simulink model "hpt_frt_full"  (R2025a)
settings: Solver=ode23tb  StartTime=0.0  StopTime=0.6  RelTol=1e-3
undefined symbols (not defined in the file or in its folder): D11, Delta
libraries: spsThreePhaseVIMeasurementLib x3, spsLinearTransformerLib x3, spsSeriesRLCBranchLib x2, spsThreePhaseSeriesRLCBranchLib x2, spsThreePhaseTransformerTwoWindingsLib x2, spsUniversalBridgeLib x2, spsIGBTLib x1, spsThreePhaseProgrammableVoltageSourceLib x1, spsThreePhaseFaultLib x1, spsThreePhaseSeriesRLCLoadLib x1, spsVoltageMeasurementLib x1, spspowerguiLib x1
settings Model: Creator=m1391  LastModifiedBy=m1391

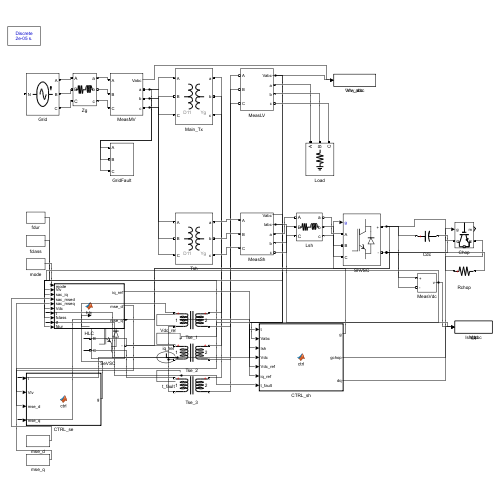
[thumbnail: Simulink's stored preview of the top-level diagram]
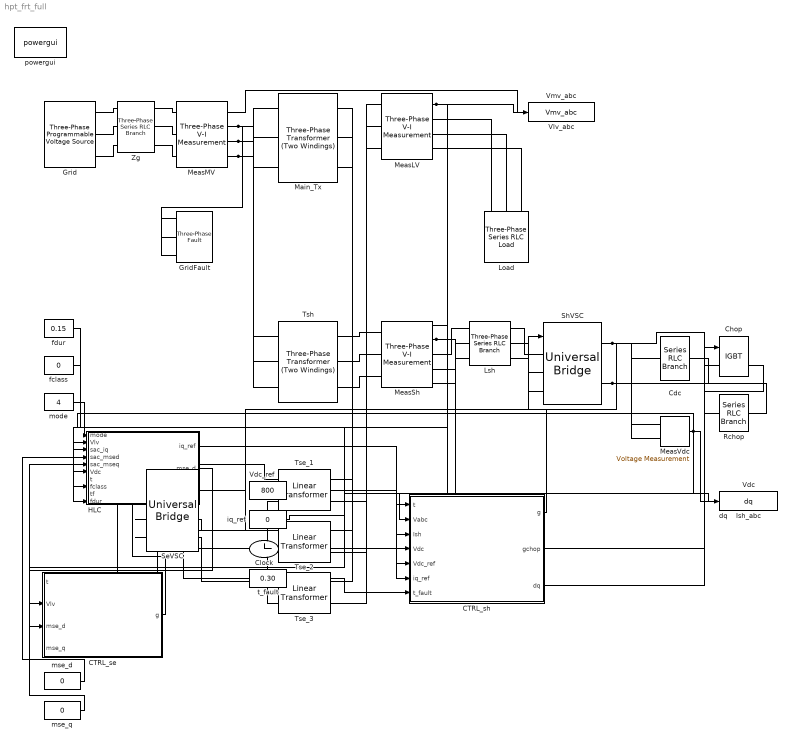
== system hpt_frt_full ==
  CTRL_se : MATLAB Function  TreatAsAtomicUnit=on
  CTRL_sh : MATLAB Function  TreatAsAtomicUnit=on
  Cdc : spsSeriesRLCBranchLib/Series RLC Branch  LConnTagsString=__new0  RConnTagsString=__new0  BranchType=C  Resistance=1  Inductance=1e-3  SetiL0=off  InitialCurrent=0  Capacitance=0.0022  Setx0=on  InitialVoltage=800  Measurements=None
  Chop : spsIGBTLib/IGBT  Ron=0.001  Lon=0  Vf=1  Tf=1e-6  Tt=2e-6  IC=0  Rs=1e5  Cs=inf  Measurements=on
  Clock : Clock
  Grid : spsThreePhaseProgrammableVoltageSourceLib/Three-Phase Programmable Voltage Source  PositiveSequence=[11250 0 50]  VariationEntity=None  VariationType=Table of time-amplitude pairs  VariationTypeAlt=Step  VariationStep=0.5  VariationRate=10  VariationMagnitude=0.3  VariationFrequency=2  VariationTiming=[1 2]  VariationPhaseA=off  Amplitudes=[1 0.8 1.2 1.0]  TimeValues=[0 0.1 0.15 0.2]  HarmonicGeneration=off  HarmonicA=[3 0.2 -25 0]  HarmonicB=[2 0.15 35 2]  Timing="[0.05  3]"  BusType=swing  Pref=0  Qref=0  Qmin=-inf  Qmax=inf
  GridFault : spsThreePhaseFaultLib/Three-Phase Fault  InitialStates=0  FaultA=off  FaultB=off  FaultC=off  GroundFault=off  SwitchTimes=[99 100]  External=off  SwitchStatus=NaN  FaultResistance=1  GroundResistance=0.01  SnubberResistance=1e6  SnubberCapacitance=inf  Measurements=None
  HLC : MATLAB Function  TreatAsAtomicUnit=on
  Ish_abc : ToWorkspace  VariableName=Ish_abc  SampleTime=2e-05
  Load : spsThreePhaseSeriesRLCLoadLib/Three-Phase Series RLC Load  LConnTagsString=A|B|C  Configuration=Y (grounded)  NominalVoltage=400  Vabc=[1e3 1e3 1e3]  Vabcp=[1e3 1e3 1e3]  NominalFrequency=50  UnbalancedPower=off  ActivePower=400000  InductivePower=0  CapacitivePower=0  Pabc=[10e3 9e3 11e3]  QLabc=[100 90 110]  QCabc=[100 90 110]  Pabcp=[10e3 9e3 11e3]  QLabcp=[100 90 110]  QCabcp=[100 90 110]  Measurements=None  LoadType=constant Z
  Lsh : spsThreePhaseSeriesRLCBranchLib/Three-Phase Series RLC Branch  LConnTagsString=A|B|C  RConnTagsString=A|B|C  BranchType=RL  Resistance=0.05  Inductance=0.003  Capacitance=1e-6  Measurements=None
  Main_Tx : spsThreePhaseTransformerTwoWindingsLib/Three-Phase Transformer (Two Windings)  Winding1Connection=Delta (D11)  Winding2Connection=Yg  CoreType=Three single-phase transformers  SetSaturation=off  Hysteresis=off  DataFile='hysteresis'  SetInitialFlux=off  Measurements=None  UNITS=pu  NominalPower=[400000,50]  Winding1=[10000,0.005,0.025]  Winding2=[400,0.005,0.025]  Rm=500  Lm=500  L0=0.5  Saturation=[ 0,0 ; 0.0024,1.2 ; 1.0,1.52 ]  InitialFluxes=[ 0.8 , -0.8 , 0.7 ]  BreakLoop=off  DiscreteSolver=Trapezoidal iterative  DataType=off  TransfoNumber=1
  MeasLV : spsThreePhaseVIMeasurementLib/Three-Phase V-I Measurement  VoltageMeasurement=phase-to-ground  SetLabelV=off  LabelV=Vabc  Vpu=off  VpuLL=off  CurrentMeasurement=no  SetLabelI=off  LabelI=Iabc  Ipu=off  Pbase=100e6  Vbase=500e3  OutputType=Complex  PhasorSimulation=off  PSBequivalent=0
  MeasMV : spsThreePhaseVIMeasurementLib/Three-Phase V-I Measurement  VoltageMeasurement=phase-to-ground  SetLabelV=off  LabelV=Vabc  Vpu=off  VpuLL=off  CurrentMeasurement=no  SetLabelI=off  LabelI=Iabc  Ipu=off  Pbase=100e6  Vbase=500e3  OutputType=Complex  PhasorSimulation=off  PSBequivalent=0
  MeasSh : spsThreePhaseVIMeasurementLib/Three-Phase V-I Measurement  VoltageMeasurement=phase-to-ground  SetLabelV=off  LabelV=Vabc  Vpu=off  VpuLL=off  CurrentMeasurement=yes  SetLabelI=off  LabelI=Iabc  Ipu=off  Pbase=100e6  Vbase=500e3  OutputType=Complex  PhasorSimulation=off  PSBequivalent=0
  MeasVdc : spsVoltageMeasurementLib/Voltage Measurement  PhasorSimulation=off  OutputType=Complex  PSBequivalent=0
  Rchop : spsSeriesRLCBranchLib/Series RLC Branch  LConnTagsString=__new0  RConnTagsString=__new0  BranchType=R  Resistance=5.3333  Inductance=1e-3  SetiL0=off  InitialCurrent=0  Capacitance=1e-6  Setx0=off  InitialVoltage=0  Measurements=None
  SeVSC : spsUniversalBridgeLib/Universal Bridge  Arms=3  SnubberResistance=1e5  SnubberCapacitance=inf  Device=IGBT / Diodes  Ron=1e-3  Lon=0  ForwardVoltages="[  0  0  ]"  ForwardVoltage=0  GTOparameters=[ 10e-6 , 20e-6 ]  IGBTparameters=[ 1e-6 , 2e-6 ]  Measurements=None  Measurements_2=None  converterType=Rectifier
  ShVSC : spsUniversalBridgeLib/Universal Bridge  Arms=3  SnubberResistance=1e5  SnubberCapacitance=inf  Device=IGBT / Diodes  Ron=1e-3  Lon=0  ForwardVoltages="[  0  0  ]"  ForwardVoltage=0  GTOparameters=[ 10e-6 , 20e-6 ]  IGBTparameters=[ 1e-6 , 2e-6 ]  Measurements=None  Measurements_2=None  converterType=Rectifier
  Tse_1 : spsLinearTransformerLib/Linear Transformer  UNITS=pu  NominalPower=[30000,50]  winding1=[400,0.002,0.03]  winding2=[46.2,0.002,0.03]  ThreeWindings=off  winding3=[ 315e3 0.002 0.08 ]  RmLm=[ 500 500 ]  Measurements=None  DataType=off
  Tse_2 : spsLinearTransformerLib/Linear Transformer  UNITS=pu  NominalPower=[30000,50]  winding1=[400,0.002,0.03]  winding2=[46.2,0.002,0.03]  ThreeWindings=off  winding3=[ 315e3 0.002 0.08 ]  RmLm=[ 500 500 ]  Measurements=None  DataType=off
  Tse_3 : spsLinearTransformerLib/Linear Transformer  UNITS=pu  NominalPower=[30000,50]  winding1=[400,0.002,0.03]  winding2=[46.2,0.002,0.03]  ThreeWindings=off  winding3=[ 315e3 0.002 0.08 ]  RmLm=[ 500 500 ]  Measurements=None  DataType=off
  Tsh : spsThreePhaseTransformerTwoWindingsLib/Three-Phase Transformer (Two Windings)  Winding1Connection=Delta (D11)  Winding2Connection=Yg  CoreType=Three single-phase transformers  SetSaturation=off  Hysteresis=off  DataFile='hysteresis'  SetInitialFlux=off  Measurements=None  UNITS=pu  NominalPower=[120000,50]  Winding1=[10000,0.005,0.02]  Winding2=[400,0.005,0.02]  Rm=500  Lm=500  L0=0.5  Saturation=[ 0,0 ; 0.0024,1.2 ; 1.0,1.52 ]  InitialFluxes=[ 0.8 , -0.8 , 0.7 ]  BreakLoop=off  DiscreteSolver=Trapezoidal iterative  DataType=off  TransfoNumber=1
  Vdc : ToWorkspace  VariableName=Vdc  SampleTime=2e-05
  Vdc_ref : Constant  Value=800
  Vlv_abc : ToWorkspace  VariableName=Vlv_abc  SampleTime=2e-05
  Vmv_abc : ToWorkspace  VariableName=Vmv_abc  SampleTime=2e-05
  Zg : spsThreePhaseSeriesRLCBranchLib/Three-Phase Series RLC Branch  LConnTagsString=A|B|C  RConnTagsString=A|B|C  BranchType=RL  Resistance=11.7851  Inductance=0.26259  Capacitance=1e-6  Measurements=None
  dq : ToWorkspace  VariableName=dq  SampleTime=2e-05
  fclass : Constant  Value=0
  fdur : Constant  Value=0.15
  iq_ref : Constant  Value=0
  mode : Constant  Value=4
  mse_d : Constant  Value=0
  mse_q : Constant  Value=0
  powergui : spspowerguiLib/powergui  Priority=1  SimulationMode=Discrete  SampleTime=2e-05  frequency=60  Iterations=50  frequencyindice=60  Pbase=100e6  ErrMax=1e-4  UnitsV=kV  UnitsW=MW  buscounter=0  FunctionMessages=off  echomessages=off  EnableUseOfTLC=off  CurrentSourceSwitches=off  DisableSnubberDevices=off  DisableRonSwitches=off  DisableVfSwitches=off  DisplayEquations=off  AutomaticDiscreteSolvers=off  SolverType=Tustin/Backward Euler (TBE)  Interpol=off  ExternalGateDelay=off  methode=off  Ts=100  x0status=blocks  SPID=on  SwTol=0  HookPort=off  NonlinearTolerance=1e-4  nMaxIteration=100  ContinueOnMaxIteration=off  RestoreLinks=warning  ResistiveCurrentMeasurement=off  Frange=[0:2:500]  Ylog=off  Xlog=on  ShowGrid=off  save=off  variable=ZData  structure=0  ZoomFFT=off  StartTime=0.0  cycles=1  DisplayStyle=1  fundamental=60  FreqAxis=off  MaxFrequency=1000  frequencyindicesteady=1  RmsSteady=1  display=off
  t_fault : Constant  Value=0.30
  wires:
  MeasMV/1 -> Vmv_abc/1
  MeasLV/1 -> Vlv_abc/1, CTRL_se/2(Vlv), HLC/2(Vlv)
  MeasSh/1 -> CTRL_sh/2(Vabc)
  MeasSh/2 -> CTRL_sh/3(Ish), Ish_abc/1
  MeasVdc/1 -> CTRL_sh/4(Vdc), Vdc/1, HLC/6(Vdc)
  Clock/1 -> CTRL_sh/1(t), CTRL_se/1(t), HLC/7(t)
  Vdc_ref/1 -> CTRL_sh/5(Vdc_ref)
  t_fault/1 -> CTRL_sh/7(t_fault), HLC/9(tf)
  CTRL_sh/1(g) -> ShVSC/1
  CTRL_sh/2(gchop) -> Chop/1
  CTRL_sh/3(dq) -> dq/1
  CTRL_se/1(g) -> SeVSC/1
  mode/1 -> HLC/1(mode)
  iq_ref/1 -> HLC/3(sac_iq)
  mse_d/1 -> HLC/4(sac_msed)
  mse_q/1 -> HLC/5(sac_mseq)
  fclass/1 -> HLC/8(fclass)
  fdur/1 -> HLC/10(fdur)
  HLC/1(iq_ref) -> CTRL_sh/6(iq_ref)
  HLC/2(mse_d) -> CTRL_se/3(mse_d)
  HLC/3(mse_q) -> CTRL_se/4(mse_q)
  connections:
  Grid/RConn1 -- Zg/LConn1
  Zg/RConn1 -- MeasMV/LConn1
  GridFault/LConn1 -- MeasMV/RConn1 -- Main_Tx/LConn1 -- Tsh/LConn1
  MeasLV/RConn1 -- Load/LConn1
  Grid/RConn2 -- Zg/LConn2
  Zg/RConn2 -- MeasMV/LConn2
  GridFault/LConn2 -- MeasMV/RConn2 -- Main_Tx/LConn2 -- Tsh/LConn2
  MeasLV/RConn2 -- Load/LConn2
  Grid/RConn3 -- Zg/LConn3
  Zg/RConn3 -- MeasMV/LConn3
  GridFault/LConn3 -- MeasMV/RConn3 -- Main_Tx/LConn3 -- Tsh/LConn3
  MeasLV/RConn3 -- Load/LConn3
  Tsh/RConn1 -- MeasSh/LConn1
  MeasSh/RConn1 -- Lsh/LConn1
  Lsh/RConn1 -- ShVSC/LConn1
  Tsh/RConn2 -- MeasSh/LConn2
  MeasSh/RConn2 -- Lsh/LConn2
  Lsh/RConn2 -- ShVSC/LConn2
  Tsh/RConn3 -- MeasSh/LConn3
  MeasSh/RConn3 -- Lsh/LConn3
  Lsh/RConn3 -- ShVSC/LConn3
  Cdc/LConn1 -- ShVSC/RConn1 -- MeasVdc/LConn1 -- Chop/LConn1 -- SeVSC/RConn1
  Cdc/RConn1 -- MeasVdc/LConn2 -- Rchop/RConn1 -- ShVSC/RConn2 -- SeVSC/RConn2
  Chop/RConn1 -- Rchop/LConn1
  Main_Tx/RConn1 -- Tse_1/RConn1
  Tse_1/RConn2 -- MeasLV/LConn1
  Main_Tx/RConn2 -- Tse_2/RConn1
  Tse_2/RConn2 -- MeasLV/LConn2
  Main_Tx/RConn3 -- Tse_3/RConn1
  Tse_3/RConn2 -- MeasLV/LConn3
  SeVSC/LConn1 -- Tse_1/LConn1
  SeVSC/LConn2 -- Tse_2/LConn1
  SeVSC/LConn3 -- Tse_3/LConn1
  Tse_2/LConn2 -- Tse_1/LConn2 -- Tse_3/LConn2

== matlab function hpt_frt_full/CTRL_se ==
  data: t input; g output; Vlv input; mse_d input; mse_q input
function g = ctrl(t, Vlv, mse_d, mse_q)
%#codegen
persistent th wint tprev
if isempty(th) || t<1e-9; th=0; wint=0; tprev=0; end
dt=t-tprev; if dt<0;dt=0;end; if dt>1e-3;dt=1e-3;end; tprev=t;
w0=2*pi*50;
Va=Vlv(1); Vb=Vlv(2); Vc=Vlv(3);
Valpha=(2/3)*(Va-0.5*Vb-0.5*Vc); Vbeta=(2/3)*(sqrt(3)/2)*(Vb-Vc);
Vd= cos(th)*Valpha+sin(th)*Vbeta; Vq=-sin(th)*Valpha+cos(th)*Vbeta;
Vm=sqrt(Vd*Vd+Vq*Vq); if Vm<50;Vm=50;end
wint=wint+1500*(Vq/Vm)*dt; if wint>150;wint=150;elseif wint<-150;wint=-150;end
w=w0+90*(Vq/Vm)+wint; th=th+w*dt; th=mod(th,2*pi);
% map SAC m_se (pu of LV phase, +/-0.2) -> VSC modulation index (+/-1): K=5
md=5*mse_d; mq=5*mse_q;
ma=md*cos(th)-mq*sin(th); mb=md*cos(th-2*pi/3)-mq*sin(th-2*pi/3); mc=md*cos(th+2*pi/3)-mq*sin(th+2*pi/3);
if ma>1;ma=1;elseif ma<-1;ma=-1;end
if mb>1;mb=1;elseif mb<-1;mb=-1;end
if mc>1;mc=1;elseif mc<-1;mc=-1;end
fc=5000; carrier=2*abs(2*(fc*t-floor(fc*t+0.5)))-1;
ga=ma>=carrier; gb=mb>=carrier; gc=mc>=carrier;
g=double([ga;~ga;gb;~gb;gc;~gc]);

== matlab function hpt_frt_full/CTRL_sh ==
  data: t input; g output; Vabc input; Ish input; Vdc input; Vdc_ref input; iq_ref input; t_fault input; gchop output; dq output
function [g, gchop, dq] = ctrl(t, Vabc, Ish, Vdc, Vdc_ref, iq_ref, t_fault)
%#codegen
persistent th wint idi iqi vdi tprev en idr
if isempty(th) || t < 1e-9
    th=0; wint=0; idi=0; iqi=0; vdi=0; tprev=0; en=0; idr=0;
end
if Vdc > 620; en = 1; end
dt = t - tprev; if dt<0; dt=0; end; if dt>1e-3; dt=1e-3; end; tprev=t;
w0 = 2*pi*50; Lsh = 3e-3; Imax = 244.949;
Va=Vabc(1); Vb=Vabc(2); Vc=Vabc(3);
Valpha=(2/3)*(Va-0.5*Vb-0.5*Vc); Vbeta=(2/3)*(sqrt(3)/2)*(Vb-Vc);
Vd =  cos(th)*Valpha + sin(th)*Vbeta;
Vq = -sin(th)*Valpha + cos(th)*Vbeta;
Vm = sqrt(Vd*Vd+Vq*Vq); if Vm<100; Vm=100; end
err = Vq/Vm;
Kp_pll=90; Ki_pll=1500;
wint = wint + Ki_pll*err*dt; if wint>150; wint=150; elseif wint<-150; wint=-150; end
w = w0 + Kp_pll*err + wint; th = th + w*dt; th = mod(th,2*pi);
Ia=Ish(1); Ib=Ish(2); Ic=Ish(3);
Ialpha=(2/3)*(Ia-0.5*Ib-0.5*Ic); Ibeta=(2/3)*(sqrt(3)/2)*(Ib-Ic);
id =  cos(th)*Ialpha + sin(th)*Ibeta;
iq = -sin(th)*Ialpha + cos(th)*Ibeta;
Kpv=0.50; Kiv=8.0; ev=(Vdc_ref-Vdc)/Vdc_ref;
vdi = vdi + Kiv*ev*dt; if vdi>1; vdi=1; elseif vdi<-1; vdi=-1; end
idtgt=(Kpv*ev+vdi)*Imax; if idtgt>0.9*Imax; idtgt=0.9*Imax; elseif idtgt<-0.9*Imax; idtgt=-0.9*Imax; end
dmax=4000*dt; ds=idtgt-idr; if ds>dmax; ds=dmax; elseif ds<-dmax; ds=-dmax; end; idr=idr+ds;
iqr=iq_ref; if iqr>Imax; iqr=Imax; elseif iqr<-Imax; iqr=-Imax; end
idm=sqrt(max(0,Imax*Imax-iqr*iqr)); if idr<-idm; idr=-idm; elseif idr>idm; idr=idm; end
Kp=2.5; Ki=150; ed=idr-id; eq=iqr-iq;
ud = Vd-(Kp*ed+idi)+w0*Lsh*iq;
uq = Vq-(Kp*eq+iqi)-w0*Lsh*id;
half=max(50,Vdc/2); md=ud/half; mq=uq/half;
ma=md*cos(th)-mq*sin(th); mb=md*cos(th-2*pi/3)-mq*sin(th-2*pi/3); mc=md*cos(th+2*pi/3)-mq*sin(th+2*pi/3);
if ma>1; ma=1; elseif ma<-1; ma=-1; end
if mb>1; mb=1; elseif mb<-1; mb=-1; end
if mc>1; mc=1; elseif mc<-1; mc=-1; end
fc=5000; carrier=2*abs(2*(fc*t-floor(fc*t+0.5)))-1;
ga=ma>=carrier; gb=mb>=carrier; gc=mc>=carrier;
g=double([ga;~ga;gb;~gb;gc;~gc]);
if en<0.5; g=zeros(6,1); idi=0; iqi=0; vdi=0; end
sat=(abs(md)>1)||(abs(mq)>1);
if ~sat; idi=idi+Ki*ed*dt; iqi=iqi+Ki*eq*dt; if idi>300;idi=300;elseif idi<-300;idi=-300;end; if iqi>300;iqi=300;elseif iqi<-300;iqi=-300;end; end
gchop = double(Vdc > 1.20*800);
dq = [id; iq; idr; iqr; Vd; Vm; th];

== matlab function hpt_frt_full/HLC ==
  data: mode input; iq_ref output; Vlv input; sac_iq input; sac_msed input; sac_mseq input; Vdc input; t input; fclass input; tf input; fdur input; mse_d output; mse_q output
% ===== INTERNAL HLC integer (mi) -> CANONICAL Mode (0-6) map (see CONTROL_MODES.md / controller_modes.m) =====
%   mi==7  -> Mode 1  Tuned fixed-law controller (strongest fixed law)
%   mi==8  -> Mode 2  One-step explicit MPC
%   mi==11 -> Mode 3  Unified SAC (single policy)
%   mi==12 -> Mode 5  Online-gated multi-expert SAC  ===== MAIN METHOD =====
%   mi==14 -> Mode 6  MPC-assisted residual SAC  (EXTENSION; NOT the main method, NOT pure SAC)
%   mi==4 dq-legacy / mi==5 Song-style / mi==6 Jia-style / mi==13 SAC-MPC hybrid / mi==10 fixed-setpoint
%        = DEPRECATED historical (no canonical 0-6 id; must not appear in papers) — see CONTROL_MODES.md §2.
% Internal integers and frt320_m{N}_* filenames kept UNCHANGED for reproducibility; canonical naming in CONTROL_MODES.md.
function [iq_ref, mse_d, mse_q] = hlc(mode, Vlv, sac_iq, sac_msed, sac_mseq, Vdc, t, fclass, tf, fdur)
%#codegen
% build-nonce 20260625-214158-605: forces fresh codegen so coder.load re-reads weight .mat files
persistent ba bb bi la vpf vnf kstep ahold onset
if isempty(ba); ba=zeros(250,1); bb=zeros(250,1); bi=1; la=zeros(3,1); vpf=1; vnf=0; kstep=int32(0); ahold=zeros(3,1); onset=-1; end
Imax=173.205; Vnom=326.599; Iact=816.497;
iq_ref=0; mse_d=0; mse_q=0;
Va=Vlv(1); Vb=Vlv(2); Vc=Vlv(3);
Valpha=(2/3)*(Va-0.5*Vb-0.5*Vc); Vbeta=(2/3)*(sqrt(3)/2)*(Vb-Vc);
Vpu=sqrt(Valpha*Valpha+Vbeta*Vbeta)/Vnom;
mi=int32(mode);
proj_en=0; if mi==int32(16); proj_en=1; mi=int32(14); end
if mi==11 || mi==12 || mi==13 || mi==14 || mi==15 || mi==17
    % ===== closed-loop SAC (11=single/Mode3, 12=online-gated 4-expert/Mode5, 15=ORACLE-gated/Mode4 ablation, 17=4-expert+residual hybrid), frt-v2 20-D obs / 3-D action / de-privileged online detector =====
    NB=250;
    Vad=ba(bi); Vbd=bb(bi); ba(bi)=Valpha; bb(bi)=Vbeta; bi=bi+1; if bi>NB; bi=1; end
    V1a=0.5*(Valpha-Vbd); V1b=0.5*(Vbeta+Vad);
    V2a=0.5*(Valpha+Vbd); V2b=0.5*(Vbeta-Vad);
    V2p=sqrt(V1a*V1a+V1b*V1b)/Vnom; V2n=sqrt(V2a*V2a+V2b*V2b)/Vnom;
    af=0.005; vpf=vpf+af*(V2p-vpf); vnf=vnf+af*(V2n-vnf); V2p=vpf; V2n=vnf;
    fc=fclass;
    if mi==11 || mi==12 || mi==13 || mi==14 || mi==17
        if V2p>1.1; fc=5; elseif V2n>0.05; fc=2; else; fc=1; end
    end
    piq=0; pmb=0;
    if V2p<0.9
        piq=1.5*(0.9-V2p); if piq>0.27; piq=0.27; end
        sgi=0.08*piq/max(0.3,V2p); fb=(Vdc/800-0.80)/0.04; if fb<0; fb=0; elseif fb>1; fb=1; end
        pmb=(0.18-sgi)/1.9; if pmb<0; pmb=0; elseif pmb>0.2; pmb=0.2; end; pmb=pmb*fb;
    elseif V2p>1.1
        piq=-1.5*(V2p-1.1); if piq<-0.27; piq=-0.27; end
        pmb=-1.5*(V2p-1.1); if pmb<-0.2; pmb=-0.2; end
    end
    if mi==13 && V2p>1.1
        % hybrid mode: HVRT domain -> analytic MPC law (mode-8 logic); LVRT -> SAC experts below
        iqp13=-1.5*(V2p-1.1); if iqp13<-0.27; iqp13=-0.27; end
        iq_ref=iqp13*Iact;
        mb13=1.5*(V2p-1.1); if mb13>0.2; mb13=0.2; end
        mse_d=mb13; mse_q=0;
    else
    kstep=kstep+int32(1); if kstep>int32(100); kstep=int32(1); end
    if kstep==int32(1)
    iqp=la(2); vdev=0.9-V2p;
    if V2p<0.9; idr=1.5*(0.9-V2p); if idr>0.3; idr=0.3; end; elseif V2p>1.1; idr=-1.5*(V2p-1.1); if idr<-0.3; idr=-0.3; end; else; idr=0; end
    iqerr=idr-iqp;
    % DE-PRIVILEGED online detector (audit #3): in_fault + elapsed from MEASURED (V2p,V2n) only,
    % NEVER the true tf/fdur (those input ports are now vestigial). Latches onset, resets on recovery.
    faulted = (V2p<0.9) || (V2p>1.1) || (V2n>0.05);
    if faulted; if onset<0; onset=t; end; else; onset=-1; end
    infault=double(faulted); elapsed=0; if faulted; elapsed=max(0,t-onset); end
    probs=zeros(6,1);
    if infault>0.5; ci=round(fc)+1; if ci<1; ci=1; elseif ci>6; ci=6; end; probs(ci)=0.92; probs(1)=probs(1)+0.08; else; probs(1)=1; end
    tfrac=elapsed*0.2/0.5; if tfrac<0; tfrac=0; elseif tfrac>1; tfrac=1; end
    obs=reshape([Vdc/800; V2p; V2n; abs(iqp); 0; 0; vdev; iqerr; iqp; probs; tfrac; infault; la(1); la(2); la(3)],20,1);
    if mi==11
        W=coder.load('sac_actor_weights.mat');
    elseif mi==14
        W=coder.load('sac_residual_weights.mat');
    elseif mi==15
        oc=round(fc);
        if oc==6; W=coder.load('sac_hvrt_asym_weights.mat');
        elseif oc==5; W=coder.load('sac_hvrt_sym_weights.mat');
        elseif oc==2; W=coder.load('sac_asym_weights.mat');
        else; W=coder.load('sac_sym_weights.mat'); end
    else
        if V2p>1.1
            if V2n>0.05; W=coder.load('sac_hvrt_asym_weights.mat'); else; W=coder.load('sac_hvrt_sym_weights.mat'); end
        elseif V2n>0.05; W=coder.load('sac_asym_weights.mat');
        else; W=coder.load('sac_sym_weights.mat'); end
    end
    W0=reshape(W.latent_pi_0_weight,256,20); b0=reshape(W.latent_pi_0_bias,256,1);
    W2=reshape(W.latent_pi_2_weight,256,256); b2=reshape(W.latent_pi_2_bias,256,1);
    W4=reshape(W.latent_pi_4_weight,256,256); b4=reshape(W.latent_pi_4_bias,256,1);
    Wm=reshape(W.mu_weight,3,256); bm=reshape(W.mu_bias,3,1);
    alo=reshape(W.act_low,3,1); ahi=reshape(W.act_high,3,1);
    h=max(0, W0*obs + b0); h=max(0, W2*h + b2); h=max(0, W4*h + b4);
    mu=Wm*h + bm; at=tanh(mu); act=alo + 0.5*(at+1).*(ahi-alo);
    if mi==17
        Wr=coder.load('sac_resexpert_weights.mat');
        r0=reshape(Wr.latent_pi_0_weight,256,20); rb0=reshape(Wr.latent_pi_0_bias,256,1);
        r2=reshape(Wr.latent_pi_2_weight,256,256); rb2=reshape(Wr.latent_pi_2_bias,256,1);
        r4=reshape(Wr.latent_pi_4_weight,256,256); rb4=reshape(Wr.latent_pi_4_bias,256,1);
        rm=reshape(Wr.mu_weight,3,256); rbm=reshape(Wr.mu_bias,3,1);
        rlo=reshape(Wr.act_low,3,1); rhi=reshape(Wr.act_high,3,1);
        hr=max(0, r0*obs + rb0); hr=max(0, r2*hr + rb2); hr=max(0, r4*hr + rb4);
        mur=rm*hr + rbm; atr=tanh(mur); actr=rlo + 0.5*(atr+1).*(rhi-rlo);
        act=act+actr;
    end
    if (mi==12 || mi==13 || mi==14 || mi==15 || mi==17) && V2p>=0.9 && V2p<=1.1 && infault<0.5; act=zeros(3,1); end
    la=act; ahold=act;
    else
    act=ahold;
    end
    if mi==14
        % residual mode: total = receding MPC prior + held residual, clipped to physical caps.
        % asym-aware iq cap (0.24): measured peak = cmd x k_2w; ODE cannot see ripple (m14-v1 lesson)
        cap14=0.27; if V2n>0.05 && V2p<0.9; cap14=0.24; end
        a1=piq+act(1); if a1>cap14; a1=cap14; elseif a1<-cap14; a1=-cap14; end
        a2=pmb+act(2); if a2>0.2; a2=0.2; elseif a2<-0.2; a2=-0.2; end
        a3=act(3); if a3>0.2; a3=0.2; elseif a3<-0.2; a3=-0.2; end
        if proj_en>0.5
            if V2p<0.9 && a1<-1e-3; a1=0; end
            if V2p>1.1 && a1>1e-3; a1=0; end
        end
        iq_ref=a1*Iact; mse_d=-a2; mse_q=-a3;
    elseif mi==17
        % 4-expert+residual hybrid: act = gated expert prior + residual (summed above). Apply the SAME
        % physical caps as mode-14 + the wrong-sign reactive dead-band (ALWAYS on = safety_projection Part-1).
        cap17=0.27; if V2n>0.05 && V2p<0.9; cap17=0.24; end
        a1=act(1); if a1>cap17; a1=cap17; elseif a1<-cap17; a1=-cap17; end
        a2=act(2); if a2>0.2; a2=0.2; elseif a2<-0.2; a2=-0.2; end
        a3=act(3); if a3>0.2; a3=0.2; elseif a3<-0.2; a3=-0.2; end
        if V2p<0.9 && a1<-1e-3; a1=0; end
        if V2p>1.1 && a1>1e-3; a1=0; end
        iq_ref=a1*Iact; mse_d=-a2; mse_q=-a3;
    else
        iq_ref=act(1)*Iact; mse_d=-act(2); mse_q=-act(3);
    end
    end
elseif mi==10
    iq_ref=sac_iq; mse_d=-sac_msed; mse_q=-sac_mseq;
else
    % dq traditional variants. All share the GB/T reactive droop (K1=1.5, cap 0.3 pu):
    if Vpu<0.9; iqp=1.5*(0.9-Vpu); if iqp>0.3; iqp=0.3; end; iq_ref=iqp*Iact;
    elseif Vpu>1.1; iqp=-1.5*(Vpu-1.1); if iqp<-0.3; iqp=-0.3; end; iq_ref=iqp*Iact;
    else; iq_ref=0; end
    if mi==8
        % week3 decision-layer one-step MPC: constrained optimum on the CALIBRATED model, receding horizon @2ms.
        % max voltage support s.t. |iq|<=0.27, Vdc_eq>=0.82 (Vdc_eq = 1 - 0.08|iq|/max(0.3,V) - 1.9*boost), |mse|<=0.2.
        % Algebraic model => closed-form optimum: series boost used UP TO the DC-budget bound (vs mode5/7 zeroing).
        if iq_ref>0.27*Iact; iq_ref=0.27*Iact; elseif iq_ref<-0.27*Iact; iq_ref=-0.27*Iact; end
        iqpu=iq_ref/Iact;
        if Vpu<0.9
            sgi=0.08*abs(iqpu)/max(0.3,Vpu);
            mb=(1.0-0.82-sgi)/1.9; if mb<0; mb=0; elseif mb>0.2; mb=0.2; end
            fb=(Vdc/800-0.80)/0.04; if fb<0; fb=0; elseif fb>1; fb=1; end
            mse_d=-mb*fb; mse_q=0;
        elseif Vpu>1.1
            mb=1.5*(Vpu-1.1); if mb>0.2; mb=0.2; end
            mse_d=mb; mse_q=0;
        else
            mse_d=0; mse_q=0;
        end
    elseif mi==7
        % Song-style + RL-backported iq headroom cap (0.27): strongest fixed-law baseline
        if iq_ref>0.27*Iact; iq_ref=0.27*Iact; elseif iq_ref<-0.27*Iact; iq_ref=-0.27*Iact; end
        mse_d=0; mse_q=0;
    elseif mi==5
        % Song-style (HPT w/o storage, lit. default): NO series action during FRT
        mse_d=0; mse_q=0;
    elseif mi==6
        % Jia-style DC-budget-aware: proportional series, linearly derated as Vdc sags
        md=-0.6*(1-Vpu); if md>0.2; md=0.2; elseif md<-0.2; md=-0.2; end
        der=(Vdc/800-0.78)/(0.95-0.78); if der<0; der=0; elseif der>1; der=1; end
        mse_d=md*der; mse_q=0;
    else
        % mode 4 (legacy baseline): fixed proportional series support
        md=-0.6*(1-Vpu); if md>0.2; md=0.2; elseif md<-0.2; md=-0.2; end
        mse_d=md; mse_q=0;
    end
end
